simulink library "SIXOSEM_T_WD_AC_MASTER"  (Simulink 8.0)
settings: Solver=ode45  StartTime=0.0  StopTime=10.0  RelTol=1e-3
libraries: cdsFilt x6, cdsRms x6, cdsTP x6, cdsEpicsOut x6, cdsEpicsIn x1
settings Model: Creator=controls  LastModifiedBy=controls

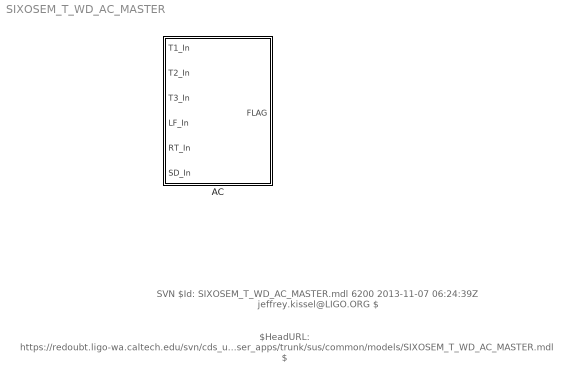
== system SIXOSEM_T_WD_AC_MASTER ==
  note: $HeadURL: https://redoubt.ligo-wa.caltech.edu/svn/cds_user_apps/trunk/sus/common/models/SIXOSEM_T_WD_AC_MASTER.mdl $
  note: SVN $Id: SIXOSEM_T_WD_AC_MASTER.mdl 6200 2013-11-07 06:24:39Z jeffrey.kissel@LIGO.ORG $
  AC : Subsystem

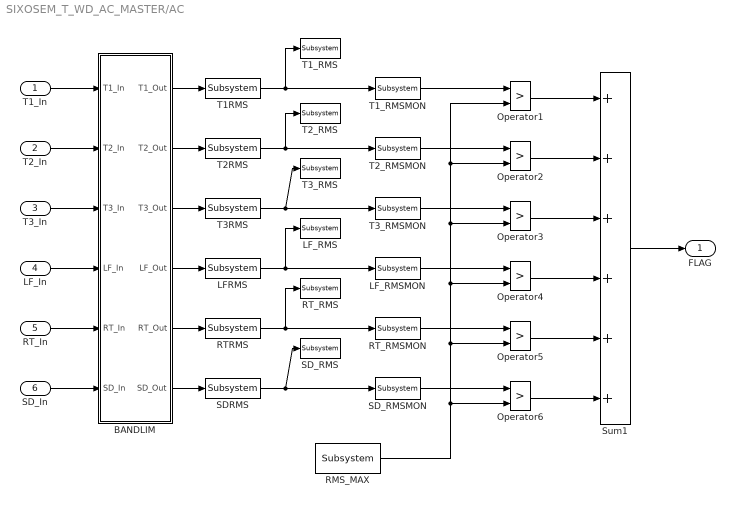
== system SIXOSEM_T_WD_AC_MASTER/AC ==
  T1_In : Inport
  T2_In : Inport  Port=2
  T3_In : Inport  Port=3
  LF_In : Inport  Port=4
  RT_In : Inport  Port=5
  SD_In : Inport  Port=6
  BANDLIM : Subsystem
  LFRMS : cdsRms/Subsystem  Tag=cdsRms  Description=|  SystemSampleTime=-1
      | Purpose:
      | Calculate an RMS based on the input signal.
      settings: AttributesFormatString=%<Tag>
  LF_RMS : cdsTP/Subsystem  Tag=Test Point  SystemSampleTime=-1
      settings: AttributesFormatString=%<Tag>
  LF_RMSMON : cdsEpicsOut/Subsystem  Tag=cdsEpicsOutput  Description=|  SystemSampleTime=-1
      | Purpose:                                          
      | Output a FE signal to an EPICS channel.           
      |                                                   
      | Operation:                                        
      | Takes input value and passes it to EPICS record.  
      |                                                   
      | Usage:                                            
      | Name the part with the desired EPICS rrecord name.
      settings: AttributesFormatString=%<Tag>
  Operator{1,3..6} (5 alike) : RelationalOperator  Operator=>  OutDataTypeStr=boolean
  Operator2 : RelationalOperator  Operator=>  OutDataTypeStr=boolean  ZeroCross=off
  RMS_MAX : cdsEpicsIn/Subsystem  Tag=cdsEpicsIn  Description=|  SystemSampleTime=-1
      | Purpose:                                                                              
      | Create an EPICS input channel connection to the FE realtime controls.                 
      |                                                                                       
      | Operation:                                                                            
      | Outputs value from an EPICS ai record. Value is floating point with a precision of 3..
      |                                                                                       
      | Usage:                                                                                
      | Name the part with the desired EPICS channel name.
      settings: AttributesFormatString=%<Tag>
  RTRMS : cdsRms/Subsystem  Tag=cdsRms  Description=|  SystemSampleTime=-1
      | Purpose:
      | Calculate an RMS based on the input signal.
      settings: AttributesFormatString=%<Tag>
  RT_RMS : cdsTP/Subsystem  Tag=Test Point  SystemSampleTime=-1
      settings: AttributesFormatString=%<Tag>
  RT_RMSMON : cdsEpicsOut/Subsystem  Tag=cdsEpicsOutput  Description=|  SystemSampleTime=-1
      | Purpose:                                          
      | Output a FE signal to an EPICS channel.           
      |                                                   
      | Operation:                                        
      | Takes input value and passes it to EPICS record.  
      |                                                   
      | Usage:                                            
      | Name the part with the desired EPICS rrecord name.
      settings: AttributesFormatString=%<Tag>
  SDRMS : cdsRms/Subsystem  Tag=cdsRms  Description=|  SystemSampleTime=-1
      | Purpose:
      | Calculate an RMS based on the input signal.
      settings: AttributesFormatString=%<Tag>
  SD_RMS : cdsTP/Subsystem  Tag=Test Point  SystemSampleTime=-1
      settings: AttributesFormatString=%<Tag>
  SD_RMSMON : cdsEpicsOut/Subsystem  Tag=cdsEpicsOutput  Description=|  SystemSampleTime=-1
      | Purpose:                                          
      | Output a FE signal to an EPICS channel.           
      |                                                   
      | Operation:                                        
      | Takes input value and passes it to EPICS record.  
      |                                                   
      | Usage:                                            
      | Name the part with the desired EPICS rrecord name.
      settings: AttributesFormatString=%<Tag>
  Sum1 : Sum  Inputs=++++++
  T1RMS : cdsRms/Subsystem  Tag=cdsRms  Description=|  SystemSampleTime=-1
      | Purpose:
      | Calculate an RMS based on the input signal.
      settings: AttributesFormatString=%<Tag>
  T1_RMS : cdsTP/Subsystem  Tag=Test Point  SystemSampleTime=-1
      settings: AttributesFormatString=%<Tag>
  T1_RMSMON : cdsEpicsOut/Subsystem  Tag=cdsEpicsOutput  Description=|  SystemSampleTime=-1
      | Purpose:                                          
      | Output a FE signal to an EPICS channel.           
      |                                                   
      | Operation:                                        
      | Takes input value and passes it to EPICS record.  
      |                                                   
      | Usage:                                            
      | Name the part with the desired EPICS rrecord name.
      settings: AttributesFormatString=%<Tag>
  T2RMS : cdsRms/Subsystem  Tag=cdsRms  Description=|  SystemSampleTime=-1
      | Purpose:
      | Calculate an RMS based on the input signal.
      settings: AttributesFormatString=%<Tag>
  T2_RMS : cdsTP/Subsystem  Tag=Test Point  SystemSampleTime=-1
      settings: AttributesFormatString=%<Tag>
  T2_RMSMON : cdsEpicsOut/Subsystem  Tag=cdsEpicsOutput  Description=|  SystemSampleTime=-1
      | Purpose:                                          
      | Output a FE signal to an EPICS channel.           
      |                                                   
      | Operation:                                        
      | Takes input value and passes it to EPICS record.  
      |                                                   
      | Usage:                                            
      | Name the part with the desired EPICS rrecord name.
      settings: AttributesFormatString=%<Tag>
  T3RMS : cdsRms/Subsystem  Tag=cdsRms  Description=|  SystemSampleTime=-1
      | Purpose:
      | Calculate an RMS based on the input signal.
      settings: AttributesFormatString=%<Tag>
  T3_RMS : cdsTP/Subsystem  Tag=Test Point  SystemSampleTime=-1
      settings: AttributesFormatString=%<Tag>
  T3_RMSMON : cdsEpicsOut/Subsystem  Tag=cdsEpicsOutput  Description=|  SystemSampleTime=-1
      | Purpose:                                          
      | Output a FE signal to an EPICS channel.           
      |                                                   
      | Operation:                                        
      | Takes input value and passes it to EPICS record.  
      |                                                   
      | Usage:                                            
      | Name the part with the desired EPICS rrecord name.
      settings: AttributesFormatString=%<Tag>
  FLAG : Outport
  wires:
  BANDLIM/6(SD_Out) -> SDRMS/1
  BANDLIM/5(RT_Out) -> RTRMS/1
  BANDLIM/4(LF_Out) -> LFRMS/1
  BANDLIM/3(T3_Out) -> T3RMS/1
  BANDLIM/2(T2_Out) -> T2RMS/1
  BANDLIM/1(T1_Out) -> T1RMS/1
  SD_In/1 -> BANDLIM/6(SD_In)
  RT_In/1 -> BANDLIM/5(RT_In)
  LF_In/1 -> BANDLIM/4(LF_In)
  T3_In/1 -> BANDLIM/3(T3_In)
  T2_In/1 -> BANDLIM/2(T2_In)
  T1_In/1 -> BANDLIM/1(T1_In)
  Operator1/1 -> Sum1/1
  Operator2/1 -> Sum1/2
  Operator3/1 -> Sum1/3
  Operator4/1 -> Sum1/4
  RMS_MAX/1 -> Operator1/2, Operator2/2, Operator3/2, Operator4/2, Operator5/2, Operator6/2
  T2RMS/1 -> T2_RMS/1, T2_RMSMON/1
  T1RMS/1 -> T1_RMS/1, T1_RMSMON/1
  T3RMS/1 -> T3_RMS/1, T3_RMSMON/1
  LFRMS/1 -> LF_RMS/1, LF_RMSMON/1
  Sum1/1 -> FLAG/1
  RTRMS/1 -> RT_RMS/1, RT_RMSMON/1
  SDRMS/1 -> SD_RMS/1, SD_RMSMON/1
  T1_RMSMON/1 -> Operator1/1
  T2_RMSMON/1 -> Operator2/1
  T3_RMSMON/1 -> Operator3/1
  LF_RMSMON/1 -> Operator4/1
  RT_RMSMON/1 -> Operator5/1
  SD_RMSMON/1 -> Operator6/1
  Operator5/1 -> Sum1/5
  Operator6/1 -> Sum1/6

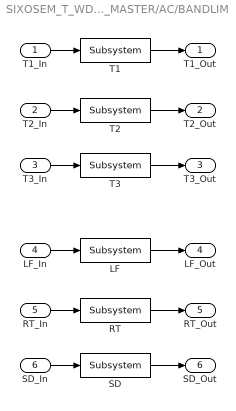
== system SIXOSEM_T_WD_AC_MASTER/AC/BANDLIM ==
  T1_In : Inport
  T2_In : Inport  Port=2
  T3_In : Inport  Port=3
  LF_In : Inport  Port=4
  RT_In : Inport  Port=5
  SD_In : Inport  Port=6
  LF : cdsFilt/Subsystem  Tag=cdsFilt  Description=|  SystemSampleTime=-1
      | Purpose:                                                                                                                                                                                                                                  
      | Standard CDS IIR filter module.                                                                                                                                                                                                           
      |                                                                                                                                                                                                                                           
      | Operation:                                                                                                                                                                                                                                
      | Consists of 10 second order section IIR filters, plus a ramped gain stage. In FE code, also provides pre-defined test points and excitation channel inputs. The filter coefficients are defined in the LIGO system using the 'foton' tool.
      |                                                                                                                                                                                                                                           
      | Usage:                                                                                                                                                                                                                                    
      | Name the part with the desired filter module name.
      settings: AttributesFormatString=%<Tag>
  RT : cdsFilt/Subsystem  Tag=cdsFilt  Description=|  SystemSampleTime=-1
      | Purpose:                                                                                                                                                                                                                                  
      | Standard CDS IIR filter module.                                                                                                                                                                                                           
      |                                                                                                                                                                                                                                           
      | Operation:                                                                                                                                                                                                                                
      | Consists of 10 second order section IIR filters, plus a ramped gain stage. In FE code, also provides pre-defined test points and excitation channel inputs. The filter coefficients are defined in the LIGO system using the 'foton' tool.
      |                                                                                                                                                                                                                                           
      | Usage:                                                                                                                                                                                                                                    
      | Name the part with the desired filter module name.
      settings: AttributesFormatString=%<Tag>
  SD : cdsFilt/Subsystem  Tag=cdsFilt  Description=|  SystemSampleTime=-1
      | Purpose:                                                                                                                                                                                                                                  
      | Standard CDS IIR filter module.                                                                                                                                                                                                           
      |                                                                                                                                                                                                                                           
      | Operation:                                                                                                                                                                                                                                
      | Consists of 10 second order section IIR filters, plus a ramped gain stage. In FE code, also provides pre-defined test points and excitation channel inputs. The filter coefficients are defined in the LIGO system using the 'foton' tool.
      |                                                                                                                                                                                                                                           
      | Usage:                                                                                                                                                                                                                                    
      | Name the part with the desired filter module name.
      settings: AttributesFormatString=%<Tag>
  T1 : cdsFilt/Subsystem  Tag=cdsFilt  Description=|  SystemSampleTime=-1
      | Purpose:                                                                                                                                                                                                                                  
      | Standard CDS IIR filter module.                                                                                                                                                                                                           
      |                                                                                                                                                                                                                                           
      | Operation:                                                                                                                                                                                                                                
      | Consists of 10 second order section IIR filters, plus a ramped gain stage. In FE code, also provides pre-defined test points and excitation channel inputs. The filter coefficients are defined in the LIGO system using the 'foton' tool.
      |                                                                                                                                                                                                                                           
      | Usage:                                                                                                                                                                                                                                    
      | Name the part with the desired filter module name.
      settings: AttributesFormatString=%<Tag>
  T2 : cdsFilt/Subsystem  Tag=cdsFilt  Description=|  SystemSampleTime=-1
      | Purpose:                                                                                                                                                                                                                                  
      | Standard CDS IIR filter module.                                                                                                                                                                                                           
      |                                                                                                                                                                                                                                           
      | Operation:                                                                                                                                                                                                                                
      | Consists of 10 second order section IIR filters, plus a ramped gain stage. In FE code, also provides pre-defined test points and excitation channel inputs. The filter coefficients are defined in the LIGO system using the 'foton' tool.
      |                                                                                                                                                                                                                                           
      | Usage:                                                                                                                                                                                                                                    
      | Name the part with the desired filter module name.
      settings: AttributesFormatString=%<Tag>
  T3 : cdsFilt/Subsystem  Tag=cdsFilt  Description=|  SystemSampleTime=-1
      | Purpose:                                                                                                                                                                                                                                  
      | Standard CDS IIR filter module.                                                                                                                                                                                                           
      |                                                                                                                                                                                                                                           
      | Operation:                                                                                                                                                                                                                                
      | Consists of 10 second order section IIR filters, plus a ramped gain stage. In FE code, also provides pre-defined test points and excitation channel inputs. The filter coefficients are defined in the LIGO system using the 'foton' tool.
      |                                                                                                                                                                                                                                           
      | Usage:                                                                                                                                                                                                                                    
      | Name the part with the desired filter module name.
      settings: AttributesFormatString=%<Tag>
  T1_Out : Outport
  T2_Out : Outport  Port=2
  T3_Out : Outport  Port=3
  LF_Out : Outport  Port=4
  RT_Out : Outport  Port=5
  SD_Out : Outport  Port=6
  wires:
  T1/1 -> T1_Out/1
  T2/1 -> T2_Out/1
  T3/1 -> T3_Out/1
  T1_In/1 -> T1/1
  T2_In/1 -> T2/1
  T3_In/1 -> T3/1
  LF/1 -> LF_Out/1
  RT/1 -> RT_Out/1
  SD/1 -> SD_Out/1
  LF_In/1 -> LF/1
  RT_In/1 -> RT/1
  SD_In/1 -> SD/1
